simulink model "gm_sampleModel1821_1_sub"  (R2023a)
settings: Solver=VariableStepAuto  StartTime=0.0  StopTime=10.0  RelTol=1e-3
libraries: hdlsllib x1, hdlmdlgenlib x1
settings Model: Creator=user1  LastModifiedBy=user1
settings OptimizationCC: BlockReduction=off  ConditionallyExecuteInputs=off
settings DebuggingCC: InheritedTsInSrcMsg=none

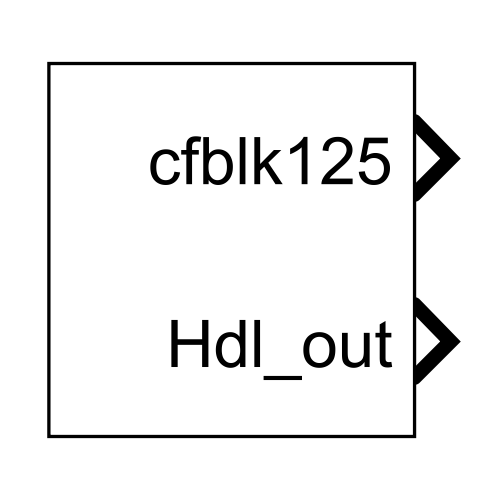
[thumbnail: Simulink's stored preview of the top-level diagram]
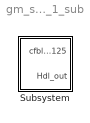
== system gm_sampleModel1821_1_sub ==
  Subsystem : Subsystem

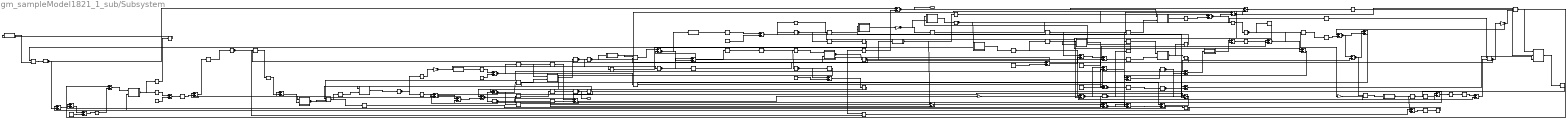
== system gm_sampleModel1821_1_sub/Subsystem ==
  Mysubsystem_10 : Subsystem
  Mysubsystem_17 : Subsystem
  Reshape{,1..10} (11 alike) : Reshape
  cfblk1 : hdlsllib/Logic and Bit Operations/Bit Concat  numInputs=2
  cfblk{10,26,43,48,65..67,82,92,98,121} (11 alike) : Signum  SampleTime=1
  cfblk{5,14,17,37,53,57,100,103,107} (9 alike) : Sum  AccumDataTypeStr=uint8  OutDataTypeStr=uint8  RndMeth=Nearest  SampleTime=1
  cfblk100_const_val : Constant  Value=0  VectorParams1D=off  OutDataTypeStr=uint8  SampleTime=1
  cfblk{7,9,18,21,25,28,33,49,55,61,63,68,77,79..81,83,93,101,105,118,122} (22 alike) : Sum  AccumDataTypeStr=uint8  OutDataTypeStr=uint8  SampleTime=1
  cfblk{13,41,45,75,102,108} (6 alike) : MinMax  OutDataTypeStr=uint8
  cfblk103_const_val : Constant  Value=0  VectorParams1D=off  OutDataTypeStr=uint8  SampleTime=1
  cfblk{58,76,87,104,112} (5 alike) : Gain  Gain="fi(0,0,8,7,\"hex\",\"80\")"  ParamDataTypeStr=fixdt(0, 8, 7)  OutDataTypeStr=uint8  SampleTime=1
  cfblk{11,23..24,27,30,40,46,51,69,95,106,110} (12 alike) : Sum  Inputs=+  OutDataTypeStr=uint8
  cfblk107_const_val : Constant  Value=0  VectorParams1D=off  OutDataTypeStr=uint8  SampleTime=1
  cfblk{31,34,47,50,52,59,88,97,113,115,124} (11 alike) : Abs  SampleTime=1  OutDataTypeStr=uint8  SaturateOnIntegerOverflow=off
  cfblk114_inst : Subsystem
  cfblk117_inst : Subsystem
  cfblk119_inst : Subsystem
  cfblk{20,29,38,42,64,72..73,91,120} (9 alike) : Sum  Inputs=+-  AccumDataTypeStr=uint8  OutDataTypeStr=uint8  SampleTime=1
  cfblk130 : Constant  OutDataTypeStr=uint8  SampleTime=1
  cfblk131 : Subsystem
  cfblk133 : Subsystem
  cfblk134 : Subsystem
  cfblk135 : Subsystem
  cfblk136 : Subsystem
  cfblk137 : Switch  Threshold=double(0)  OutDataTypeStr=uint8  SampleTime=1  SaturateOnIntegerOverflow=off  InputSameDT=off
  cfblk139 : Switch  Threshold=double(0)  OutDataTypeStr=uint8  SampleTime=1  SaturateOnIntegerOverflow=off  InputSameDT=off
  cfblk140 : Switch  Threshold=double(0)  OutDataTypeStr=uint8  SampleTime=1  SaturateOnIntegerOverflow=off  InputSameDT=off
  cfblk{141..145,147..159,161} (19 alike) : Delay  DelayLength=double(2)  InitialCondition=0  SampleTime=1
  cfblk14_const_val : Constant  Value=0  VectorParams1D=off  OutDataTypeStr=uint8  SampleTime=1
  cfblk{162..165,168} (5 alike) : DataTypeConversion  OutDataTypeStr=fixdt(0,8,0)
  cfblk166 : DataTypeConversion  OutDataTypeStr=uint8  SampleTime=1  SaturateOnIntegerOverflow=off  RndMeth=Floor
  cfblk167 : DataTypeConversion  OutDataTypeStr=uint8  SampleTime=1  SaturateOnIntegerOverflow=off  RndMeth=Floor
  cfblk17_const_val : Constant  Value=0  VectorParams1D=off  OutDataTypeStr=uint8  SampleTime=1
  cfblk{6,19,22,44} (4 alike) : Product  Inputs=*/  OutDataTypeStr=uint8  RndMeth=Zero  SaturateOnIntegerOverflow=on  SampleTime=1
  cfblk2 : RelationalOperator  Operator=<=  OutDataTypeStr=boolean  SampleTime=1  InputSameDT=off
  cfblk3 : Subsystem  mask(Compare To Zero){relop=<=, OutDataTypeStr=uint8, ZeroCross=on}
      mask prompts: relop "Simulink:masks:Operator_MP"; OutDataTypeStr "Simulink:masks:OutputDataType_MP"; ZeroCross "Simulink:masks:EnableZerocrossingDetection_MP"
      mask help: Simulink:masks:CompareToZero_MD
      mask init:
      | OutDataTypeStr = 'uint8';
      | ZeroCross = 'on';
      | blkName = 'sampleModel1821_1_sub/Subsystem/cfblk3';
      | relop = '<=';
      | setValue = 'fixdt(0, 8)';
      mask TypeOptions relop: == | ~= | < | <= | >= | >
      mask TypeOptions OutDataTypeStr: Simulink:masks:uint8 | Simulink:masks:boolean
      mask Callback ZeroCross: sl('zeroCrossEnable', gcbh);
      mask Display: disp([relop,' 0'])
  cfblk32 : Sum  AccumDataTypeStr=uint32  OutDataTypeStr=uint8  SampleTime=1
  cfblk36_inst : Subsystem
  cfblk37_const_val : Constant  Value=0  VectorParams1D=off  OutDataTypeStr=uint8  SampleTime=1
  cfblk39_inst : Subsystem
  cfblk4 : hdlmdlgenlib/Buffer
  cfblk53_const_val : Constant  Value=0  VectorParams1D=off  OutDataTypeStr=uint8  SampleTime=1
  cfblk56_inst : Subsystem
  cfblk57_const_val : Constant  Value=0  VectorParams1D=off  OutDataTypeStr=uint8  SampleTime=1
  cfblk5_const_val : Constant  Value=0  VectorParams1D=off  OutDataTypeStr=uint8  SampleTime=1
  cfblk62_inst : Subsystem
  cfblk74_inst : Subsystem
  cfblk78_inst : Subsystem
  cfblk86_inst : Subsystem
  cfblk99_inst : Subsystem
  cfblk125 : Outport  OutDataTypeStr=uint8  SampleTime=1  VectorParamsAs1DForOutWhenUnconnected=off
  Hdl_out : Outport  Port=2  OutDataTypeStr=uint8  SampleTime=1
  wires:
  Mysubsystem_10/1(Out1) -> cfblk1/2
  Mysubsystem_17/1(Out1) -> cfblk154/1
  cfblk1/1 -> cfblk167/1
  cfblk10/1 -> cfblk77/1, cfblk3/1(u)
  cfblk100/1 -> cfblk21/2
  cfblk101/1 -> cfblk61/2, cfblk131/1(In1)
  cfblk102/1 -> cfblk99_inst/2(in2), Reshape1/1, cfblk44/2
  cfblk103/1 -> cfblk112/1
  cfblk104/1 -> Reshape2/1, cfblk119_inst/2(in2)
  cfblk105/1 -> cfblk17/1
  cfblk106/1 -> cfblk18/2, cfblk137/2
  cfblk107/1 -> cfblk50/1
  cfblk108/1 -> cfblk144/1
  cfblk11/1 -> cfblk4/1
  cfblk110/1 -> cfblk74_inst/2(in2)
  Reshape/1 -> cfblk102/1
  cfblk112/1 -> cfblk28/1
  cfblk113/1 -> cfblk26/1, cfblk27/1
  cfblk114_inst/1(out1) -> cfblk104/1
  cfblk115/1 -> cfblk103/1
  cfblk117_inst/1(out1) -> cfblk113/1
  cfblk118/1 -> cfblk9/2
  cfblk119_inst/1(out1) -> cfblk66/1
  cfblk120/1 -> cfblk6/2
  cfblk121/1 -> cfblk93/1, cfblk52/1
  cfblk122/1 -> Mysubsystem_17/3(In3)
  cfblk124/1 -> cfblk43/1
  cfblk13/1 -> cfblk64/2, cfblk36_inst/2(in2)
  cfblk130/1 -> cfblk25/1, cfblk21/1
  cfblk131/1(Out1) -> cfblk23/1
  cfblk133/1(Out1) -> Reshape10/1
  cfblk134/1(Out1) -> cfblk33/2, cfblk19/1
  cfblk135/1(Out1) -> cfblk33/1
  cfblk136/1(Out1) -> cfblk55/2, cfblk121/1
  cfblk137/1 -> cfblk105/1
  cfblk139/1 -> cfblk48/1
  cfblk14/1 -> cfblk145/1
  cfblk140/1 -> cfblk118/2
  cfblk141/1 -> cfblk120/1
  cfblk142/1 -> cfblk83/2
  cfblk143/1 -> cfblk73/2
  cfblk144/1 -> cfblk72/2
  cfblk145/1 -> cfblk32/2
  cfblk147/1 -> cfblk77/2
  cfblk148/1 -> cfblk81/1
  cfblk149/1 -> cfblk80/2
  Reshape1/1 -> cfblk142/1
  cfblk150/1 -> cfblk20/2
  cfblk151/1 -> cfblk117_inst/2(in2)
  cfblk152/1 -> cfblk162/1
  cfblk153/1 -> cfblk6/1
  cfblk154/1 -> cfblk78_inst/1(in1)
  cfblk155/1 -> cfblk56_inst/2(in2)
  cfblk156/1 -> cfblk119_inst/1(in1)
  cfblk157/1 -> cfblk114_inst/1(in1)
  cfblk158/1 -> cfblk19/2
  cfblk159/1 -> cfblk168/1
  Reshape2/1 -> cfblk153/1
  cfblk161/1 -> cfblk93/2
  cfblk162/1 -> cfblk165/1, Hdl_out/1
  cfblk163/1 -> cfblk152/1
  cfblk164/1 -> cfblk59/1, cfblk161/1
  cfblk165/1 -> cfblk86_inst/1(in1)
  cfblk166/1 -> cfblk86_inst/2(in2)
  cfblk167/1 -> cfblk73/1, cfblk49/2
  cfblk168/1 -> cfblk1/1
  cfblk17/1 -> Reshape7/1
  cfblk18/1 -> cfblk135/1(In1)
  cfblk19/1 -> cfblk101/1
  cfblk2/1 -> cfblk32/1, cfblk166/1, cfblk51/1
  cfblk20/1 -> cfblk83/1, cfblk38/2
  cfblk21/1 -> cfblk107/1
  cfblk22/1 -> cfblk68/1, Mysubsystem_17/1(In1)
  cfblk23/1 -> cfblk37/1
  cfblk24/1 -> Reshape5/1, cfblk69/1
  cfblk25/1 -> cfblk139/2, cfblk22/1
  cfblk26/1 -> cfblk9/1, cfblk134/1(In1)
  cfblk27/1 -> Reshape9/1, cfblk61/1
  cfblk28/1 -> Reshape4/1
  cfblk29/1 -> cfblk151/1, cfblk150/1
  cfblk3/1(y) -> cfblk140/1, cfblk148/1
  cfblk30/1 -> cfblk42/1, cfblk159/1
  cfblk31/1 -> cfblk76/1, cfblk40/1
  cfblk32/1 -> Reshape/1
  cfblk33/1 -> cfblk147/1
  cfblk34/1 -> cfblk122/1, cfblk156/1
  Reshape3/1 -> cfblk14/1
  cfblk36_inst/1(out1) -> cfblk57/1
  cfblk37/1 -> cfblk88/1, cfblk137/3, cfblk30/1
  cfblk38/1 -> cfblk67/1, cfblk29/2, cfblk140/3, cfblk137/1
  cfblk39_inst/1(out1) -> cfblk45/1
  cfblk4/1 -> cfblk18/1, cfblk122/2
  cfblk40/1 -> cfblk36_inst/1(in1)
  cfblk41/1 -> cfblk24/1
  cfblk42/1 -> cfblk91/1
  cfblk43/1 -> Mysubsystem_10/1(In1)
  cfblk44/1 -> cfblk55/1
  cfblk45/1 -> cfblk64/1, cfblk13/1
  cfblk46/1 -> cfblk117_inst/1(in1), cfblk115/1
  cfblk47/1 -> Reshape8/1
  cfblk48/1 -> Mysubsystem_17/2(In2)
  cfblk49/1 -> cfblk105/2
  cfblk5/1 -> cfblk149/1, cfblk46/1
  cfblk50/1 -> cfblk74_inst/1(in1)
  cfblk51/1 -> cfblk7/1
  cfblk52/1 -> cfblk28/2
  cfblk53/1 -> cfblk97/1
  Reshape4/1 -> cfblk141/1
  cfblk55/1 -> cfblk47/1
  cfblk56_inst/1(out1) -> cfblk65/1
  cfblk57/1 -> cfblk155/1, cfblk11/1
  cfblk58/1 -> cfblk72/1, cfblk22/2
  cfblk59/1 -> cfblk87/1
  cfblk6/1 -> cfblk101/2, cfblk58/1
  cfblk61/1 -> cfblk41/1
  cfblk62_inst/1(out1) -> Reshape3/1, cfblk124/1
  cfblk63/1 -> cfblk110/1
  cfblk64/1 -> cfblk7/2, cfblk63/1, cfblk34/1
  cfblk65/1 -> cfblk81/2
  cfblk66/1 -> cfblk39_inst/1(in1), cfblk139/3
  cfblk67/1 -> cfblk163/1, cfblk140/2
  cfblk68/1 -> cfblk62_inst/1(in1)
  cfblk69/1 -> cfblk99_inst/1(in1)
  cfblk7/1 -> cfblk91/2, cfblk118/1
  Reshape5/1 -> cfblk53/1, cfblk95/1
  Reshape6/1 -> cfblk136/1(In1)
  cfblk72/1 -> cfblk80/1, cfblk79/2
  cfblk73/1 -> cfblk56_inst/1(in1), cfblk139/1, cfblk125/1
  cfblk74_inst/1(out1) -> cfblk158/1, cfblk157/1
  cfblk75/1 -> cfblk114_inst/2(in2)
  cfblk76/1 -> cfblk120/2
  cfblk77/1 -> cfblk42/2, cfblk108/1
  cfblk78_inst/1(out1) -> cfblk63/2, cfblk2/2
  cfblk79/1 -> cfblk2/1
  cfblk80/1 -> cfblk79/1, Reshape6/1
  cfblk81/1 -> cfblk82/1, cfblk25/2
  cfblk82/1 -> cfblk31/1
  cfblk83/1 -> cfblk78_inst/2(in2)
  Reshape7/1 -> cfblk68/2
  Reshape8/1 -> cfblk62_inst/2(in2)
  cfblk86_inst/1(out1) -> cfblk164/1
  cfblk87/1 -> cfblk98/1, cfblk133/1(In1)
  cfblk88/1 -> cfblk75/1
  Reshape9/1 -> cfblk100/1
  cfblk9/1 -> cfblk92/1
  Reshape10/1 -> cfblk5/1
  cfblk91/1 -> cfblk106/1
  cfblk92/1 -> cfblk49/1
  cfblk93/1 -> cfblk20/1
  cfblk95/1 -> cfblk38/1
  cfblk97/1 -> cfblk29/1
  cfblk98/1 -> cfblk39_inst/2(in2)
  cfblk99_inst/1(out1) -> cfblk10/1, cfblk44/1, cfblk143/1
  cfblk100_const_val/1 -> cfblk100/2
  cfblk103_const_val/1 -> cfblk103/2
  cfblk107_const_val/1 -> cfblk107/2
  cfblk14_const_val/1 -> cfblk14/2
  cfblk17_const_val/1 -> cfblk17/2
  cfblk37_const_val/1 -> cfblk37/2
  cfblk5_const_val/1 -> cfblk5/2
  cfblk53_const_val/1 -> cfblk53/2
  cfblk57_const_val/1 -> cfblk57/2

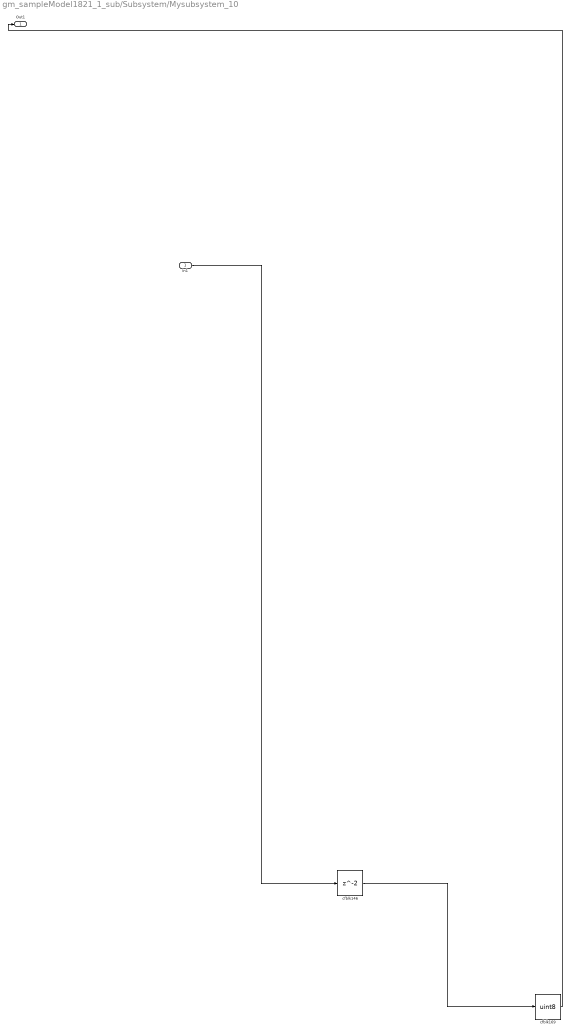
== system gm_sampleModel1821_1_sub/Subsystem/Mysubsystem_10 ==
  In1 : Inport  OutDataTypeStr=uint8  PortDimensions=1  SampleTime=1
  cfblk146 : Delay  SampleTime=1
  cfblk169 : DataTypeConversion  OutDataTypeStr=uint8  SaturateOnIntegerOverflow=off  RndMeth=Floor
  Out1 : Outport  SampleTime=1
  wires:
  In1/1 -> cfblk146/1
  cfblk146/1 -> cfblk169/1
  cfblk169/1 -> Out1/1

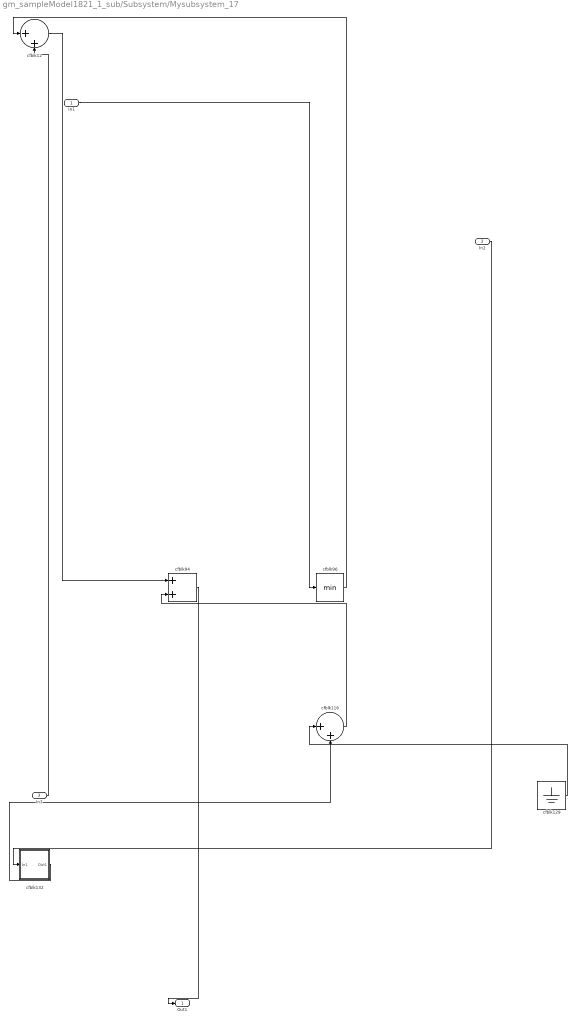
== system gm_sampleModel1821_1_sub/Subsystem/Mysubsystem_17 ==
  In1 : Inport  OutDataTypeStr=uint8  PortDimensions=1  SampleTime=1
  In2 : Inport  Port=2  OutDataTypeStr=uint8  PortDimensions=1  SampleTime=1
  In3 : Inport  Port=3  OutDataTypeStr=uint8  PortDimensions=1  SampleTime=1
  cfblk116 : Sum  Inputs=|++
  cfblk12 : Sum  Inputs=|++
  cfblk129 : Ground
  cfblk132 : Subsystem
  cfblk94 : Sum
  cfblk96 : MinMax
  Out1 : Outport  SampleTime=1
  wires:
  In1/1 -> cfblk96/1
  In2/1 -> cfblk132/1(In1)
  In3/1 -> cfblk12/2
  cfblk116/1 -> cfblk94/2
  cfblk12/1 -> cfblk94/1
  cfblk129/1 -> cfblk116/1
  cfblk132/1(Out1) -> cfblk116/2
  cfblk94/1 -> Out1/1
  cfblk96/1 -> cfblk12/1

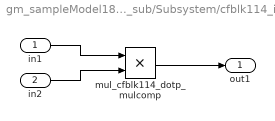
== system gm_sampleModel1821_1_sub/Subsystem/cfblk114_inst ==
  in1 : Inport  OutDataTypeStr=uint8  SampleTime=1
  in2 : Inport  Port=2  OutDataTypeStr=uint8  SampleTime=1
  mul_cfblk114_dotp_mulcomp : Product  Inputs=**  OutDataTypeStr=uint8  SampleTime=1
  out1 : Outport  OutDataTypeStr=uint8  SampleTime=1
  wires:
  in1/1 -> mul_cfblk114_dotp_mulcomp/1
  in2/1 -> mul_cfblk114_dotp_mulcomp/2
  mul_cfblk114_dotp_mulcomp/1 -> out1/1

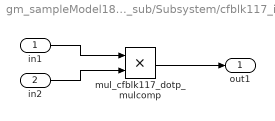
== system gm_sampleModel1821_1_sub/Subsystem/cfblk117_inst ==
  in1 : Inport  OutDataTypeStr=uint8  SampleTime=1
  in2 : Inport  Port=2  OutDataTypeStr=uint8  SampleTime=1
  mul_cfblk117_dotp_mulcomp : Product  Inputs=**  OutDataTypeStr=uint8  SampleTime=1
  out1 : Outport  OutDataTypeStr=uint8  SampleTime=1
  wires:
  in1/1 -> mul_cfblk117_dotp_mulcomp/1
  in2/1 -> mul_cfblk117_dotp_mulcomp/2
  mul_cfblk117_dotp_mulcomp/1 -> out1/1

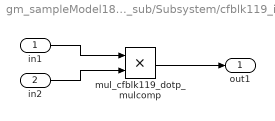
== system gm_sampleModel1821_1_sub/Subsystem/cfblk119_inst ==
  in1 : Inport  OutDataTypeStr=uint8  SampleTime=1
  in2 : Inport  Port=2  OutDataTypeStr=uint8  SampleTime=1
  mul_cfblk119_dotp_mulcomp : Product  Inputs=**  OutDataTypeStr=uint8  SampleTime=1
  out1 : Outport  OutDataTypeStr=uint8  SampleTime=1
  wires:
  in1/1 -> mul_cfblk119_dotp_mulcomp/1
  in2/1 -> mul_cfblk119_dotp_mulcomp/2
  mul_cfblk119_dotp_mulcomp/1 -> out1/1

== system gm_sampleModel1821_1_sub/Subsystem/cfblk131 ==
  In1 : Inport  OutDataTypeStr=uint8  PortDimensions=1  SampleTime=1
  Out1 : Outport  SampleTime=1
  wires:
  In1/1 -> Out1/1

== system gm_sampleModel1821_1_sub/Subsystem/cfblk133 ==
  In1 : Inport  OutDataTypeStr=uint8  PortDimensions=1  SampleTime=1
  Out1 : Outport  SampleTime=1
  wires:
  In1/1 -> Out1/1

== system gm_sampleModel1821_1_sub/Subsystem/cfblk134 ==
  In1 : Inport  OutDataTypeStr=uint8  PortDimensions=1  SampleTime=1
  Out1 : Outport  SampleTime=1
  wires:
  In1/1 -> Out1/1

== system gm_sampleModel1821_1_sub/Subsystem/cfblk135 ==
  In1 : Inport  OutDataTypeStr=uint8  PortDimensions=1  SampleTime=1
  Out1 : Outport  SampleTime=1
  wires:
  In1/1 -> Out1/1

== system gm_sampleModel1821_1_sub/Subsystem/cfblk136 ==
  In1 : Inport  OutDataTypeStr=uint8  PortDimensions=1  SampleTime=1
  Out1 : Outport  SampleTime=1
  wires:
  In1/1 -> Out1/1

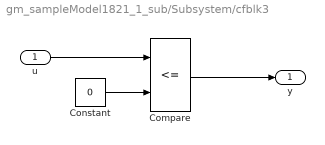
== system gm_sampleModel1821_1_sub/Subsystem/cfblk3 ==
  u : Inport  OutDataTypeStr=uint8  SampleTime=1
  Compare : RelationalOperator  Operator=<=  OutDataTypeStr=fixdt(0, 8)
  Constant : Constant  DisableCoverage=on  Value=0  OutDataTypeStr=Inherit: Inherit via back propagation  SampleTime=-1  PreserveConstantTs=on
  y : Outport  SampleTime=1
  wires:
  u/1 -> Compare/1
  Compare/1 -> y/1
  Constant/1 -> Compare/2

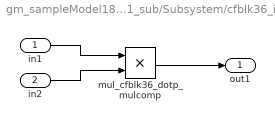
== system gm_sampleModel1821_1_sub/Subsystem/cfblk36_inst ==
  in1 : Inport  OutDataTypeStr=uint8  SampleTime=1
  in2 : Inport  Port=2  OutDataTypeStr=uint8  SampleTime=1
  mul_cfblk36_dotp_mulcomp : Product  Inputs=**  OutDataTypeStr=uint8  SampleTime=1
  out1 : Outport  OutDataTypeStr=uint8  SampleTime=1
  wires:
  in1/1 -> mul_cfblk36_dotp_mulcomp/1
  in2/1 -> mul_cfblk36_dotp_mulcomp/2
  mul_cfblk36_dotp_mulcomp/1 -> out1/1

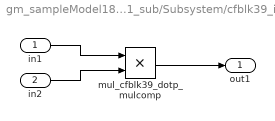
== system gm_sampleModel1821_1_sub/Subsystem/cfblk39_inst ==
  in1 : Inport  OutDataTypeStr=uint8  SampleTime=1
  in2 : Inport  Port=2  OutDataTypeStr=uint8  SampleTime=1
  mul_cfblk39_dotp_mulcomp : Product  Inputs=**  OutDataTypeStr=uint8  SampleTime=1
  out1 : Outport  OutDataTypeStr=uint8  SampleTime=1
  wires:
  in1/1 -> mul_cfblk39_dotp_mulcomp/1
  in2/1 -> mul_cfblk39_dotp_mulcomp/2
  mul_cfblk39_dotp_mulcomp/1 -> out1/1

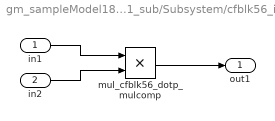
== system gm_sampleModel1821_1_sub/Subsystem/cfblk56_inst ==
  in1 : Inport  OutDataTypeStr=uint8  SampleTime=1
  in2 : Inport  Port=2  OutDataTypeStr=uint8  SampleTime=1
  mul_cfblk56_dotp_mulcomp : Product  Inputs=**  OutDataTypeStr=uint8  SampleTime=1
  out1 : Outport  OutDataTypeStr=uint8  SampleTime=1
  wires:
  in1/1 -> mul_cfblk56_dotp_mulcomp/1
  in2/1 -> mul_cfblk56_dotp_mulcomp/2
  mul_cfblk56_dotp_mulcomp/1 -> out1/1

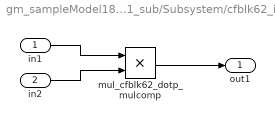
== system gm_sampleModel1821_1_sub/Subsystem/cfblk62_inst ==
  in1 : Inport  OutDataTypeStr=uint8  SampleTime=1
  in2 : Inport  Port=2  OutDataTypeStr=uint8  SampleTime=1
  mul_cfblk62_dotp_mulcomp : Product  Inputs=**  OutDataTypeStr=uint8  SampleTime=1
  out1 : Outport  OutDataTypeStr=uint8  SampleTime=1
  wires:
  in1/1 -> mul_cfblk62_dotp_mulcomp/1
  in2/1 -> mul_cfblk62_dotp_mulcomp/2
  mul_cfblk62_dotp_mulcomp/1 -> out1/1

== system gm_sampleModel1821_1_sub/Subsystem/cfblk74_inst ==
  in1 : Inport  OutDataTypeStr=uint8  SampleTime=1
  in2 : Inport  Port=2  OutDataTypeStr=uint8  SampleTime=1
  mul_cfblk74_dotp_mulcomp : Product  Inputs=**  OutDataTypeStr=uint8  SampleTime=1
  out1 : Outport  OutDataTypeStr=uint8  SampleTime=1
  wires:
  in1/1 -> mul_cfblk74_dotp_mulcomp/1
  in2/1 -> mul_cfblk74_dotp_mulcomp/2
  mul_cfblk74_dotp_mulcomp/1 -> out1/1

== system gm_sampleModel1821_1_sub/Subsystem/cfblk78_inst ==
  in1 : Inport  OutDataTypeStr=uint8  SampleTime=1
  in2 : Inport  Port=2  OutDataTypeStr=uint8  SampleTime=1
  mul_cfblk78_dotp_mulcomp : Product  Inputs=**  OutDataTypeStr=uint8  SampleTime=1
  out1 : Outport  OutDataTypeStr=uint8  SampleTime=1
  wires:
  in1/1 -> mul_cfblk78_dotp_mulcomp/1
  in2/1 -> mul_cfblk78_dotp_mulcomp/2
  mul_cfblk78_dotp_mulcomp/1 -> out1/1

== system gm_sampleModel1821_1_sub/Subsystem/cfblk86_inst ==
  in1 : Inport  OutDataTypeStr=uint8  SampleTime=1
  in2 : Inport  Port=2  OutDataTypeStr=uint8  SampleTime=1
  mul_cfblk86_dotp_mulcomp : Product  Inputs=**  OutDataTypeStr=uint8  SampleTime=1
  out1 : Outport  OutDataTypeStr=uint8  SampleTime=1
  wires:
  in1/1 -> mul_cfblk86_dotp_mulcomp/1
  in2/1 -> mul_cfblk86_dotp_mulcomp/2
  mul_cfblk86_dotp_mulcomp/1 -> out1/1

== system gm_sampleModel1821_1_sub/Subsystem/cfblk99_inst ==
  in1 : Inport  OutDataTypeStr=uint8  SampleTime=1
  in2 : Inport  Port=2  OutDataTypeStr=uint8  SampleTime=1
  mul_cfblk99_dotp_mulcomp : Product  Inputs=**  OutDataTypeStr=uint8  SampleTime=1
  out1 : Outport  OutDataTypeStr=uint8  SampleTime=1
  wires:
  in1/1 -> mul_cfblk99_dotp_mulcomp/1
  in2/1 -> mul_cfblk99_dotp_mulcomp/2
  mul_cfblk99_dotp_mulcomp/1 -> out1/1

== system gm_sampleModel1821_1_sub/Subsystem/Mysubsystem_17/cfblk132 ==
  In1 : Inport  OutDataTypeStr=uint8  PortDimensions=1  SampleTime=1
  Out1 : Outport  SampleTime=1
  wires:
  In1/1 -> Out1/1
